simulink model "BicyclePeterCorkeP2P"  (R2021a)
settings: Solver=VariableStepAuto  StartTime=0.0  StopTime=30  RelTol=1e-3
values from neighbouring files (symbols this model uses):
  accelLim = 1    [BicyclePeterCorkeLineFollowSetup.m]    (also in BicyclePeterCorkePathFollowSetup.m; BicyclePeterCorkePoseReachSetup.m)
  initCoord = [8 0 pi/2]    [BicyclePeterCorkeLineFollowSetup.m]    (also in BicyclePeterCorkePathFollowSetup.m = [0 0 -pi/2])
  speedLim = 1    [BicyclePeterCorkeLineFollowSetup.m]    (also in BicyclePeterCorkePathFollowSetup.m; BicyclePeterCorkePoseReachSetup.m)
  steerLim = 1    [BicyclePeterCorkeLineFollowSetup.m]    (also in BicyclePeterCorkePathFollowSetup.m; BicyclePeterCorkePoseReachSetup.m)
  wheelBase = 1    [BicyclePeterCorkeLineFollowSetup.m]    (also in BicyclePeterCorkePathFollowSetup.m; BicyclePeterCorkePoseReachSetup.m)
undefined symbols (not defined in the file or in its folder): goalCoord
libraries: simulink x2
settings Model: Creator=guyot  LastModifiedBy=User

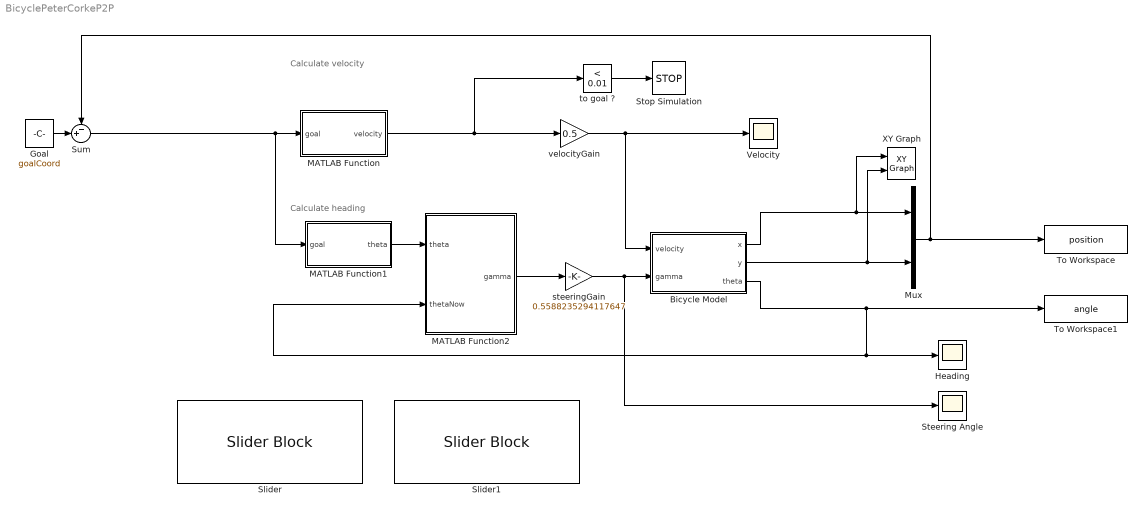
== system BicyclePeterCorkeP2P ==
  note: Calculate heading
  note: Calculate velocity
  Bicycle Model : Subsystem
  Goal : Constant  Value=goalCoord
  Heading : Scope
  MATLAB Function : MATLAB Function  TreatAsAtomicUnit=on
  MATLAB Function1 : MATLAB Function  TreatAsAtomicUnit=on
  MATLAB Function2 : MATLAB Function  TreatAsAtomicUnit=on
  Mux : Mux  Inputs=2
  Slider : SliderBlock  ScaleMax=2
  Slider1 : SliderBlock  ScaleMax=5
  Steering Angle : Scope
  Stop Simulation : Stop
  Sum : Sum  Inputs=-+|
  To Workspace : ToWorkspace  VariableName=position  SaveFormat=Timeseries  SampleTime=-1
  To Workspace1 : ToWorkspace  VariableName=angle  SaveFormat=Timeseries  SampleTime=-1
  Velocity : Scope
  XY Graph : simulink/Sinks/XY Graph  xmin=-2  xmax=10  ymin=-2  ymax=10  st=-1
  steeringGain : Gain  Gain=0.5588235294117647
  to goal ? : simulink/Logic and Bit Operations/Compare To Constant  relop=<  const=0.01  OutDataTypeStr=boolean
  velocityGain : Gain  Gain=0.5
  wires:
  Goal/1 -> Sum/2
  MATLAB Function/1(velocity) -> to goal ?/1, velocityGain/1
  velocityGain/1 -> Bicycle Model/1(velocity), Velocity/1
  MATLAB Function1/1(theta) -> MATLAB Function2/1(theta)
  MATLAB Function2/1(gamma) -> steeringGain/1
  steeringGain/1 -> Steering Angle/1, Bicycle Model/2(gamma)
  to goal ?/1 -> Stop Simulation/1
  Bicycle Model/1(x) -> Mux/1, XY Graph/1
  Bicycle Model/2(y) -> XY Graph/2, Mux/2
  Sum/1 -> MATLAB Function1/1(goal), MATLAB Function/1(goal)
  Bicycle Model/3(theta) -> To Workspace1/1, MATLAB Function2/2(thetaNow), Heading/1
  Mux/1 -> To Workspace/1, Sum/1

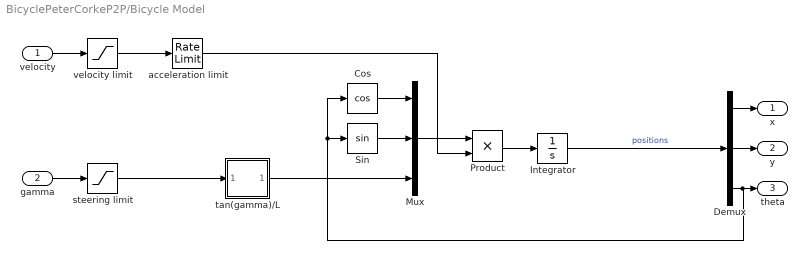
== system BicyclePeterCorkeP2P/Bicycle Model ==
  velocity : Inport
  gamma : Inport  Port=2
  Cos : Trigonometry  Operator=cos
  Demux : Demux  Outputs=3
  Integrator : Integrator  InitialCondition=initCoord
  Mux : Mux  Inputs=3
  Product : Product
  Sin : Trigonometry
  acceleration limit : RateLimiter  RisingSlewLimit=accelLim  FallingSlewLimit=-accelLim  SampleTimeMode=inherited
  steering limit : Saturate  UpperLimit=steerLim  LowerLimit=-steerLim
  tan(gamma)/L : Subsystem
  velocity limit : Saturate  UpperLimit=speedLim  LowerLimit=-speedLim
  x : Outport
  y : Outport  Port=2
  theta : Outport  Port=3
  wires:
  velocity/1 -> velocity limit/1
  velocity limit/1 -> acceleration limit/1
  gamma/1 -> steering limit/1
  steering limit/1 -> tan(gamma)/L/1(In1)
  tan(gamma)/L/1(Out1) -> Mux/3
  Mux/1 -> Product/1
  acceleration limit/1 -> Product/2
  Product/1 -> Integrator/1
  Integrator/1 -> Demux/1  "positions"
  Demux/3 -> Cos/1, Sin/1, theta/1
  Demux/1 -> x/1
  Demux/2 -> y/1
  Cos/1 -> Mux/1
  Sin/1 -> Mux/2

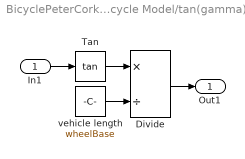
== system BicyclePeterCorkeP2P/Bicycle Model/tan(gamma)//L ==
  In1 : Inport
  Divide : Product  Inputs=*/
  Tan : Trigonometry  Operator=tan
  vehicle length : Constant  Value=wheelBase
  Out1 : Outport
  wires:
  Tan/1 -> Divide/1
  vehicle length/1 -> Divide/2
  In1/1 -> Tan/1
  Divide/1 -> Out1/1

== matlab function BicyclePeterCorkeP2P/MATLAB Function ==
  data: goal input; velocity output
function velocity = speedGoal(goal)

velocity = sqrt(goal(1)^2+goal(2)^2);

== matlab function BicyclePeterCorkeP2P/MATLAB Function2 ==
  data: theta input; gamma output; thetaNow input
function gamma = gammaGoal(theta, thetaNow)

gamma = angdiff(thetaNow, theta);

== matlab function BicyclePeterCorkeP2P/MATLAB Function1 ==
  data: goal input; theta output
function theta = goalAngle(goal)

theta = atan2(goal(2),goal(1));
